simulink model "ProcessNetworkSimulation"  (R2015b)
settings: Solver=VariableStepAuto  StartTime=0.0  StopTime=1000.0  RelTol=1e-3
libraries: simulink x1, simeventslib x1
(part 17 of 21)

== system ProcessNetworkSimulation/Process_97 ==
  IN_Job : PathCombiner  NumberInputPorts=29
  OUT_Job : OutputSwitch  NumberOutputPorts=30  SwitchingCriterion=From attribute  AttributeName=outputFlowNode
  Process : Subsystem
  IN_Job_1 : PMIOPort  Port=1  Side=Left
  IN_Job_2 : PMIOPort  Port=2  Side=Left
  IN_Job_3 : PMIOPort  Port=3  Side=Left
  IN_Job_4 : PMIOPort  Port=4  Side=Left
  IN_Job_5 : PMIOPort  Port=5  Side=Left
  IN_Job_6 : PMIOPort  Port=6  Side=Left
  IN_Job_7 : PMIOPort  Port=7  Side=Left
  IN_Job_8 : PMIOPort  Port=8  Side=Left
  IN_Job_9 : PMIOPort  Port=9  Side=Left
  IN_Job_10 : PMIOPort  Port=10  Side=Left
  IN_Job_11 : PMIOPort  Port=11  Side=Left
  IN_Job_12 : PMIOPort  Port=12  Side=Left
  IN_Job_13 : PMIOPort  Port=13  Side=Left
  IN_Job_14 : PMIOPort  Port=14  Side=Left
  IN_Job_15 : PMIOPort  Port=15  Side=Left
  IN_Job_16 : PMIOPort  Port=16  Side=Left
  IN_Job_17 : PMIOPort  Port=17  Side=Left
  IN_Job_18 : PMIOPort  Port=18  Side=Left
  IN_Job_19 : PMIOPort  Port=19  Side=Left
  IN_Job_20 : PMIOPort  Port=20  Side=Left
  IN_Job_21 : PMIOPort  Port=21  Side=Left
  IN_Job_22 : PMIOPort  Port=22  Side=Left
  IN_Job_23 : PMIOPort  Port=23  Side=Left
  IN_Job_24 : PMIOPort  Port=24  Side=Left
  IN_Job_25 : PMIOPort  Port=25  Side=Left
  IN_Job_26 : PMIOPort  Port=26  Side=Left
  IN_Job_27 : PMIOPort  Port=27  Side=Left
  IN_Job_28 : PMIOPort  Port=28  Side=Left
  IN_Job_29 : PMIOPort  Port=29  Side=Left
  OUT_Job_1 : PMIOPort  Port=30  Side=Right
  OUT_Job_2 : PMIOPort  Port=31  Side=Right
  OUT_Job_3 : PMIOPort  Port=32  Side=Right
  OUT_Job_4 : PMIOPort  Port=33  Side=Right
  OUT_Job_5 : PMIOPort  Port=34  Side=Right
  OUT_Job_6 : PMIOPort  Port=35  Side=Right
  OUT_Job_7 : PMIOPort  Port=36  Side=Right
  OUT_Job_8 : PMIOPort  Port=37  Side=Right
  OUT_Job_9 : PMIOPort  Port=38  Side=Right
  OUT_Job_10 : PMIOPort  Port=39  Side=Right
  OUT_Job_11 : PMIOPort  Port=40  Side=Right
  OUT_Job_12 : PMIOPort  Port=41  Side=Right
  OUT_Job_13 : PMIOPort  Port=42  Side=Right
  OUT_Job_14 : PMIOPort  Port=43  Side=Right
  OUT_Job_15 : PMIOPort  Port=44  Side=Right
  OUT_Job_16 : PMIOPort  Port=45  Side=Right
  OUT_Job_17 : PMIOPort  Port=46  Side=Right
  OUT_Job_18 : PMIOPort  Port=47  Side=Right
  OUT_Job_19 : PMIOPort  Port=48  Side=Right
  OUT_Job_20 : PMIOPort  Port=49  Side=Right
  OUT_Job_21 : PMIOPort  Port=50  Side=Right
  OUT_Job_22 : PMIOPort  Port=51  Side=Right
  OUT_Job_23 : PMIOPort  Port=52  Side=Right
  OUT_Job_24 : PMIOPort  Port=53  Side=Right
  OUT_Job_25 : PMIOPort  Port=54  Side=Right
  OUT_Job_26 : PMIOPort  Port=55  Side=Right
  OUT_Job_27 : PMIOPort  Port=56  Side=Right
  OUT_Job_28 : PMIOPort  Port=57  Side=Right
  OUT_Job_29 : PMIOPort  Port=58  Side=Right
  OUT_Job_30 : PMIOPort  Port=59  Side=Right
  connections:
  OUT_Job/LConn1 -- Process/RConn1
  IN_Job/RConn1 -- Process/LConn1
  IN_Job/LConn1 -- IN_Job_1/RConn1
  IN_Job/LConn2 -- IN_Job_2/RConn1
  IN_Job/LConn3 -- IN_Job_3/RConn1
  IN_Job/LConn4 -- IN_Job_4/RConn1
  IN_Job/LConn5 -- IN_Job_5/RConn1
  IN_Job/LConn6 -- IN_Job_6/RConn1
  IN_Job/LConn7 -- IN_Job_7/RConn1
  IN_Job/LConn8 -- IN_Job_8/RConn1
  IN_Job/LConn9 -- IN_Job_9/RConn1
  IN_Job/LConn10 -- IN_Job_10/RConn1
  IN_Job/LConn11 -- IN_Job_11/RConn1
  IN_Job/LConn12 -- IN_Job_12/RConn1
  IN_Job/LConn13 -- IN_Job_13/RConn1
  IN_Job/LConn14 -- IN_Job_14/RConn1
  IN_Job/LConn15 -- IN_Job_15/RConn1
  IN_Job/LConn16 -- IN_Job_16/RConn1
  IN_Job/LConn17 -- IN_Job_17/RConn1
  IN_Job/LConn18 -- IN_Job_18/RConn1
  IN_Job/LConn19 -- IN_Job_19/RConn1
  IN_Job/LConn20 -- IN_Job_20/RConn1
  IN_Job/LConn21 -- IN_Job_21/RConn1
  IN_Job/LConn22 -- IN_Job_22/RConn1
  IN_Job/LConn23 -- IN_Job_23/RConn1
  IN_Job/LConn24 -- IN_Job_24/RConn1
  IN_Job/LConn25 -- IN_Job_25/RConn1
  IN_Job/LConn26 -- IN_Job_26/RConn1
  IN_Job/LConn27 -- IN_Job_27/RConn1
  IN_Job/LConn28 -- IN_Job_28/RConn1
  IN_Job/LConn29 -- IN_Job_29/RConn1
  OUT_Job/RConn1 -- OUT_Job_1/RConn1
  OUT_Job/RConn2 -- OUT_Job_2/RConn1
  OUT_Job/RConn3 -- OUT_Job_3/RConn1
  OUT_Job/RConn4 -- OUT_Job_4/RConn1
  OUT_Job/RConn5 -- OUT_Job_5/RConn1
  OUT_Job/RConn6 -- OUT_Job_6/RConn1
  OUT_Job/RConn7 -- OUT_Job_7/RConn1
  OUT_Job/RConn8 -- OUT_Job_8/RConn1
  OUT_Job/RConn9 -- OUT_Job_9/RConn1
  OUT_Job/RConn10 -- OUT_Job_10/RConn1
  OUT_Job/RConn11 -- OUT_Job_11/RConn1
  OUT_Job/RConn12 -- OUT_Job_12/RConn1
  OUT_Job/RConn13 -- OUT_Job_13/RConn1
  OUT_Job/RConn14 -- OUT_Job_14/RConn1
  OUT_Job/RConn15 -- OUT_Job_15/RConn1
  OUT_Job/RConn16 -- OUT_Job_16/RConn1
  OUT_Job/RConn17 -- OUT_Job_17/RConn1
  OUT_Job/RConn18 -- OUT_Job_18/RConn1
  OUT_Job/RConn19 -- OUT_Job_19/RConn1
  OUT_Job/RConn20 -- OUT_Job_20/RConn1
  OUT_Job/RConn21 -- OUT_Job_21/RConn1
  OUT_Job/RConn22 -- OUT_Job_22/RConn1
  OUT_Job/RConn23 -- OUT_Job_23/RConn1
  OUT_Job/RConn24 -- OUT_Job_24/RConn1
  OUT_Job/RConn25 -- OUT_Job_25/RConn1
  OUT_Job/RConn26 -- OUT_Job_26/RConn1
  OUT_Job/RConn27 -- OUT_Job_27/RConn1
  OUT_Job/RConn28 -- OUT_Job_28/RConn1
  OUT_Job/RConn29 -- OUT_Job_29/RConn1
  OUT_Job/RConn30 -- OUT_Job_30/RConn1

== system ProcessNetworkSimulation/Process_98 ==
  IN_Job : PathCombiner  NumberInputPorts=42
  OUT_Job : OutputSwitch  NumberOutputPorts=37  SwitchingCriterion=From attribute  AttributeName=outputFlowNode
  Process : Subsystem
  IN_Job_1 : PMIOPort  Port=1  Side=Left
  IN_Job_2 : PMIOPort  Port=2  Side=Left
  IN_Job_3 : PMIOPort  Port=3  Side=Left
  IN_Job_4 : PMIOPort  Port=4  Side=Left
  IN_Job_5 : PMIOPort  Port=5  Side=Left
  IN_Job_6 : PMIOPort  Port=6  Side=Left
  IN_Job_7 : PMIOPort  Port=7  Side=Left
  IN_Job_8 : PMIOPort  Port=8  Side=Left
  IN_Job_9 : PMIOPort  Port=9  Side=Left
  IN_Job_10 : PMIOPort  Port=10  Side=Left
  IN_Job_11 : PMIOPort  Port=11  Side=Left
  IN_Job_12 : PMIOPort  Port=12  Side=Left
  IN_Job_13 : PMIOPort  Port=13  Side=Left
  IN_Job_14 : PMIOPort  Port=14  Side=Left
  IN_Job_15 : PMIOPort  Port=15  Side=Left
  IN_Job_16 : PMIOPort  Port=16  Side=Left
  IN_Job_17 : PMIOPort  Port=17  Side=Left
  IN_Job_18 : PMIOPort  Port=18  Side=Left
  IN_Job_19 : PMIOPort  Port=19  Side=Left
  IN_Job_20 : PMIOPort  Port=20  Side=Left
  IN_Job_21 : PMIOPort  Port=21  Side=Left
  IN_Job_22 : PMIOPort  Port=22  Side=Left
  IN_Job_23 : PMIOPort  Port=23  Side=Left
  IN_Job_24 : PMIOPort  Port=24  Side=Left
  IN_Job_25 : PMIOPort  Port=25  Side=Left
  IN_Job_26 : PMIOPort  Port=26  Side=Left
  IN_Job_27 : PMIOPort  Port=27  Side=Left
  IN_Job_28 : PMIOPort  Port=28  Side=Left
  IN_Job_29 : PMIOPort  Port=29  Side=Left
  IN_Job_30 : PMIOPort  Port=30  Side=Left
  IN_Job_31 : PMIOPort  Port=31  Side=Left
  IN_Job_32 : PMIOPort  Port=32  Side=Left
  IN_Job_33 : PMIOPort  Port=33  Side=Left
  IN_Job_34 : PMIOPort  Port=34  Side=Left
  IN_Job_35 : PMIOPort  Port=35  Side=Left
  IN_Job_36 : PMIOPort  Port=36  Side=Left
  IN_Job_37 : PMIOPort  Port=37  Side=Left
  IN_Job_38 : PMIOPort  Port=38  Side=Left
  IN_Job_39 : PMIOPort  Port=39  Side=Left
  IN_Job_40 : PMIOPort  Port=40  Side=Left
  IN_Job_41 : PMIOPort  Port=41  Side=Left
  IN_Job_42 : PMIOPort  Port=42  Side=Left
  OUT_Job_1 : PMIOPort  Port=43  Side=Right
  OUT_Job_2 : PMIOPort  Port=44  Side=Right
  OUT_Job_3 : PMIOPort  Port=45  Side=Right
  OUT_Job_4 : PMIOPort  Port=46  Side=Right
  OUT_Job_5 : PMIOPort  Port=47  Side=Right
  OUT_Job_6 : PMIOPort  Port=48  Side=Right
  OUT_Job_7 : PMIOPort  Port=49  Side=Right
  OUT_Job_8 : PMIOPort  Port=50  Side=Right
  OUT_Job_9 : PMIOPort  Port=51  Side=Right
  OUT_Job_10 : PMIOPort  Port=52  Side=Right
  OUT_Job_11 : PMIOPort  Port=53  Side=Right
  OUT_Job_12 : PMIOPort  Port=54  Side=Right
  OUT_Job_13 : PMIOPort  Port=55  Side=Right
  OUT_Job_14 : PMIOPort  Port=56  Side=Right
  OUT_Job_15 : PMIOPort  Port=57  Side=Right
  OUT_Job_16 : PMIOPort  Port=58  Side=Right
  OUT_Job_17 : PMIOPort  Port=59  Side=Right
  OUT_Job_18 : PMIOPort  Port=60  Side=Right
  OUT_Job_19 : PMIOPort  Port=61  Side=Right
  OUT_Job_20 : PMIOPort  Port=62  Side=Right
  OUT_Job_21 : PMIOPort  Port=63  Side=Right
  OUT_Job_22 : PMIOPort  Port=64  Side=Right
  OUT_Job_23 : PMIOPort  Port=65  Side=Right
  OUT_Job_24 : PMIOPort  Port=66  Side=Right
  OUT_Job_25 : PMIOPort  Port=67  Side=Right
  OUT_Job_26 : PMIOPort  Port=68  Side=Right
  OUT_Job_27 : PMIOPort  Port=69  Side=Right
  OUT_Job_28 : PMIOPort  Port=70  Side=Right
  OUT_Job_29 : PMIOPort  Port=71  Side=Right
  OUT_Job_30 : PMIOPort  Port=72  Side=Right
  OUT_Job_31 : PMIOPort  Port=73  Side=Right
  OUT_Job_32 : PMIOPort  Port=74  Side=Right
  OUT_Job_33 : PMIOPort  Port=75  Side=Right
  OUT_Job_34 : PMIOPort  Port=76  Side=Right
  OUT_Job_35 : PMIOPort  Port=77  Side=Right
  OUT_Job_36 : PMIOPort  Port=78  Side=Right
  OUT_Job_37 : PMIOPort  Port=79  Side=Right
  connections:
  OUT_Job/LConn1 -- Process/RConn1
  IN_Job/RConn1 -- Process/LConn1
  IN_Job/LConn1 -- IN_Job_1/RConn1
  IN_Job/LConn2 -- IN_Job_2/RConn1
  IN_Job/LConn3 -- IN_Job_3/RConn1
  IN_Job/LConn4 -- IN_Job_4/RConn1
  IN_Job/LConn5 -- IN_Job_5/RConn1
  IN_Job/LConn6 -- IN_Job_6/RConn1
  IN_Job/LConn7 -- IN_Job_7/RConn1
  IN_Job/LConn8 -- IN_Job_8/RConn1
  IN_Job/LConn9 -- IN_Job_9/RConn1
  IN_Job/LConn10 -- IN_Job_10/RConn1
  IN_Job/LConn11 -- IN_Job_11/RConn1
  IN_Job/LConn12 -- IN_Job_12/RConn1
  IN_Job/LConn13 -- IN_Job_13/RConn1
  IN_Job/LConn14 -- IN_Job_14/RConn1
  IN_Job/LConn15 -- IN_Job_15/RConn1
  IN_Job/LConn16 -- IN_Job_16/RConn1
  IN_Job/LConn17 -- IN_Job_17/RConn1
  IN_Job/LConn18 -- IN_Job_18/RConn1
  IN_Job/LConn19 -- IN_Job_19/RConn1
  IN_Job/LConn20 -- IN_Job_20/RConn1
  IN_Job/LConn21 -- IN_Job_21/RConn1
  IN_Job/LConn22 -- IN_Job_22/RConn1
  IN_Job/LConn23 -- IN_Job_23/RConn1
  IN_Job/LConn24 -- IN_Job_24/RConn1
  IN_Job/LConn25 -- IN_Job_25/RConn1
  IN_Job/LConn26 -- IN_Job_26/RConn1
  IN_Job/LConn27 -- IN_Job_27/RConn1
  IN_Job/LConn28 -- IN_Job_28/RConn1
  IN_Job/LConn29 -- IN_Job_29/RConn1
  IN_Job/LConn30 -- IN_Job_30/RConn1
  IN_Job/LConn31 -- IN_Job_31/RConn1
  IN_Job/LConn32 -- IN_Job_32/RConn1
  IN_Job/LConn33 -- IN_Job_33/RConn1
  IN_Job/LConn34 -- IN_Job_34/RConn1
  IN_Job/LConn35 -- IN_Job_35/RConn1
  IN_Job/LConn36 -- IN_Job_36/RConn1
  IN_Job/LConn37 -- IN_Job_37/RConn1
  IN_Job/LConn38 -- IN_Job_38/RConn1
  IN_Job/LConn39 -- IN_Job_39/RConn1
  IN_Job/LConn40 -- IN_Job_40/RConn1
  IN_Job/LConn41 -- IN_Job_41/RConn1
  IN_Job/LConn42 -- IN_Job_42/RConn1
  OUT_Job/RConn1 -- OUT_Job_1/RConn1
  OUT_Job/RConn2 -- OUT_Job_2/RConn1
  OUT_Job/RConn3 -- OUT_Job_3/RConn1
  OUT_Job/RConn4 -- OUT_Job_4/RConn1
  OUT_Job/RConn5 -- OUT_Job_5/RConn1
  OUT_Job/RConn6 -- OUT_Job_6/RConn1
  OUT_Job/RConn7 -- OUT_Job_7/RConn1
  OUT_Job/RConn8 -- OUT_Job_8/RConn1
  OUT_Job/RConn9 -- OUT_Job_9/RConn1
  OUT_Job/RConn10 -- OUT_Job_10/RConn1
  OUT_Job/RConn11 -- OUT_Job_11/RConn1
  OUT_Job/RConn12 -- OUT_Job_12/RConn1
  OUT_Job/RConn13 -- OUT_Job_13/RConn1
  OUT_Job/RConn14 -- OUT_Job_14/RConn1
  OUT_Job/RConn15 -- OUT_Job_15/RConn1
  OUT_Job/RConn16 -- OUT_Job_16/RConn1
  OUT_Job/RConn17 -- OUT_Job_17/RConn1
  OUT_Job/RConn18 -- OUT_Job_18/RConn1
  OUT_Job/RConn19 -- OUT_Job_19/RConn1
  OUT_Job/RConn20 -- OUT_Job_20/RConn1
  OUT_Job/RConn21 -- OUT_Job_21/RConn1
  OUT_Job/RConn22 -- OUT_Job_22/RConn1
  OUT_Job/RConn23 -- OUT_Job_23/RConn1
  OUT_Job/RConn24 -- OUT_Job_24/RConn1
  OUT_Job/RConn25 -- OUT_Job_25/RConn1
  OUT_Job/RConn26 -- OUT_Job_26/RConn1
  OUT_Job/RConn27 -- OUT_Job_27/RConn1
  OUT_Job/RConn28 -- OUT_Job_28/RConn1
  OUT_Job/RConn29 -- OUT_Job_29/RConn1
  OUT_Job/RConn30 -- OUT_Job_30/RConn1
  OUT_Job/RConn31 -- OUT_Job_31/RConn1
  OUT_Job/RConn32 -- OUT_Job_32/RConn1
  OUT_Job/RConn33 -- OUT_Job_33/RConn1
  OUT_Job/RConn34 -- OUT_Job_34/RConn1
  OUT_Job/RConn35 -- OUT_Job_35/RConn1
  OUT_Job/RConn36 -- OUT_Job_36/RConn1
  OUT_Job/RConn37 -- OUT_Job_37/RConn1

== system ProcessNetworkSimulation/Process_99 ==
  IN_Job : PathCombiner  NumberInputPorts=46
  OUT_Job : OutputSwitch  NumberOutputPorts=40  SwitchingCriterion=From attribute  AttributeName=outputFlowNode
  Process : Subsystem
  IN_Job_1 : PMIOPort  Port=1  Side=Left
  IN_Job_2 : PMIOPort  Port=2  Side=Left
  IN_Job_3 : PMIOPort  Port=3  Side=Left
  IN_Job_4 : PMIOPort  Port=4  Side=Left
  IN_Job_5 : PMIOPort  Port=5  Side=Left
  IN_Job_6 : PMIOPort  Port=6  Side=Left
  IN_Job_7 : PMIOPort  Port=7  Side=Left
  IN_Job_8 : PMIOPort  Port=8  Side=Left
  IN_Job_9 : PMIOPort  Port=9  Side=Left
  IN_Job_10 : PMIOPort  Port=10  Side=Left
  IN_Job_11 : PMIOPort  Port=11  Side=Left
  IN_Job_12 : PMIOPort  Port=12  Side=Left
  IN_Job_13 : PMIOPort  Port=13  Side=Left
  IN_Job_14 : PMIOPort  Port=14  Side=Left
  IN_Job_15 : PMIOPort  Port=15  Side=Left
  IN_Job_16 : PMIOPort  Port=16  Side=Left
  IN_Job_17 : PMIOPort  Port=17  Side=Left
  IN_Job_18 : PMIOPort  Port=18  Side=Left
  IN_Job_19 : PMIOPort  Port=19  Side=Left
  IN_Job_20 : PMIOPort  Port=20  Side=Left
  IN_Job_21 : PMIOPort  Port=21  Side=Left
  IN_Job_22 : PMIOPort  Port=22  Side=Left
  IN_Job_23 : PMIOPort  Port=23  Side=Left
  IN_Job_24 : PMIOPort  Port=24  Side=Left
  IN_Job_25 : PMIOPort  Port=25  Side=Left
  IN_Job_26 : PMIOPort  Port=26  Side=Left
  IN_Job_27 : PMIOPort  Port=27  Side=Left
  IN_Job_28 : PMIOPort  Port=28  Side=Left
  IN_Job_29 : PMIOPort  Port=29  Side=Left
  IN_Job_30 : PMIOPort  Port=30  Side=Left
  IN_Job_31 : PMIOPort  Port=31  Side=Left
  IN_Job_32 : PMIOPort  Port=32  Side=Left
  IN_Job_33 : PMIOPort  Port=33  Side=Left
  IN_Job_34 : PMIOPort  Port=34  Side=Left
  IN_Job_35 : PMIOPort  Port=35  Side=Left
  IN_Job_36 : PMIOPort  Port=36  Side=Left
  IN_Job_37 : PMIOPort  Port=37  Side=Left
  IN_Job_38 : PMIOPort  Port=38  Side=Left
  IN_Job_39 : PMIOPort  Port=39  Side=Left
  IN_Job_40 : PMIOPort  Port=40  Side=Left
  IN_Job_41 : PMIOPort  Port=41  Side=Left
  IN_Job_42 : PMIOPort  Port=42  Side=Left
  IN_Job_43 : PMIOPort  Port=43  Side=Left
  IN_Job_44 : PMIOPort  Port=44  Side=Left
  IN_Job_45 : PMIOPort  Port=45  Side=Left
  IN_Job_46 : PMIOPort  Port=46  Side=Left
  OUT_Job_1 : PMIOPort  Port=47  Side=Right
  OUT_Job_2 : PMIOPort  Port=48  Side=Right
  OUT_Job_3 : PMIOPort  Port=49  Side=Right
  OUT_Job_4 : PMIOPort  Port=50  Side=Right
  OUT_Job_5 : PMIOPort  Port=51  Side=Right
  OUT_Job_6 : PMIOPort  Port=52  Side=Right
  OUT_Job_7 : PMIOPort  Port=53  Side=Right
  OUT_Job_8 : PMIOPort  Port=54  Side=Right
  OUT_Job_9 : PMIOPort  Port=55  Side=Right
  OUT_Job_10 : PMIOPort  Port=56  Side=Right
  OUT_Job_11 : PMIOPort  Port=57  Side=Right
  OUT_Job_12 : PMIOPort  Port=58  Side=Right
  OUT_Job_13 : PMIOPort  Port=59  Side=Right
  OUT_Job_14 : PMIOPort  Port=60  Side=Right
  OUT_Job_15 : PMIOPort  Port=61  Side=Right
  OUT_Job_16 : PMIOPort  Port=62  Side=Right
  OUT_Job_17 : PMIOPort  Port=63  Side=Right
  OUT_Job_18 : PMIOPort  Port=64  Side=Right
  OUT_Job_19 : PMIOPort  Port=65  Side=Right
  OUT_Job_20 : PMIOPort  Port=66  Side=Right
  OUT_Job_21 : PMIOPort  Port=67  Side=Right
  OUT_Job_22 : PMIOPort  Port=68  Side=Right
  OUT_Job_23 : PMIOPort  Port=69  Side=Right
  OUT_Job_24 : PMIOPort  Port=70  Side=Right
  OUT_Job_25 : PMIOPort  Port=71  Side=Right
  OUT_Job_26 : PMIOPort  Port=72  Side=Right
  OUT_Job_27 : PMIOPort  Port=73  Side=Right
  OUT_Job_28 : PMIOPort  Port=74  Side=Right
  OUT_Job_29 : PMIOPort  Port=75  Side=Right
  OUT_Job_30 : PMIOPort  Port=76  Side=Right
  OUT_Job_31 : PMIOPort  Port=77  Side=Right
  OUT_Job_32 : PMIOPort  Port=78  Side=Right
  OUT_Job_33 : PMIOPort  Port=79  Side=Right
  OUT_Job_34 : PMIOPort  Port=80  Side=Right
  OUT_Job_35 : PMIOPort  Port=81  Side=Right
  OUT_Job_36 : PMIOPort  Port=82  Side=Right
  OUT_Job_37 : PMIOPort  Port=83  Side=Right
  OUT_Job_38 : PMIOPort  Port=84  Side=Right
  OUT_Job_39 : PMIOPort  Port=85  Side=Right
  OUT_Job_40 : PMIOPort  Port=86  Side=Right
  connections:
  OUT_Job/LConn1 -- Process/RConn1
  IN_Job/RConn1 -- Process/LConn1
  IN_Job/LConn1 -- IN_Job_1/RConn1
  IN_Job/LConn2 -- IN_Job_2/RConn1
  IN_Job/LConn3 -- IN_Job_3/RConn1
  IN_Job/LConn4 -- IN_Job_4/RConn1
  IN_Job/LConn5 -- IN_Job_5/RConn1
  IN_Job/LConn6 -- IN_Job_6/RConn1
  IN_Job/LConn7 -- IN_Job_7/RConn1
  IN_Job/LConn8 -- IN_Job_8/RConn1
  IN_Job/LConn9 -- IN_Job_9/RConn1
  IN_Job/LConn10 -- IN_Job_10/RConn1
  IN_Job/LConn11 -- IN_Job_11/RConn1
  IN_Job/LConn12 -- IN_Job_12/RConn1
  IN_Job/LConn13 -- IN_Job_13/RConn1
  IN_Job/LConn14 -- IN_Job_14/RConn1
  IN_Job/LConn15 -- IN_Job_15/RConn1
  IN_Job/LConn16 -- IN_Job_16/RConn1
  IN_Job/LConn17 -- IN_Job_17/RConn1
  IN_Job/LConn18 -- IN_Job_18/RConn1
  IN_Job/LConn19 -- IN_Job_19/RConn1
  IN_Job/LConn20 -- IN_Job_20/RConn1
  IN_Job/LConn21 -- IN_Job_21/RConn1
  IN_Job/LConn22 -- IN_Job_22/RConn1
  IN_Job/LConn23 -- IN_Job_23/RConn1
  IN_Job/LConn24 -- IN_Job_24/RConn1
  IN_Job/LConn25 -- IN_Job_25/RConn1
  IN_Job/LConn26 -- IN_Job_26/RConn1
  IN_Job/LConn27 -- IN_Job_27/RConn1
  IN_Job/LConn28 -- IN_Job_28/RConn1
  IN_Job/LConn29 -- IN_Job_29/RConn1
  IN_Job/LConn30 -- IN_Job_30/RConn1
  IN_Job/LConn31 -- IN_Job_31/RConn1
  IN_Job/LConn32 -- IN_Job_32/RConn1
  IN_Job/LConn33 -- IN_Job_33/RConn1
  IN_Job/LConn34 -- IN_Job_34/RConn1
  IN_Job/LConn35 -- IN_Job_35/RConn1
  IN_Job/LConn36 -- IN_Job_36/RConn1
  IN_Job/LConn37 -- IN_Job_37/RConn1
  IN_Job/LConn38 -- IN_Job_38/RConn1
  IN_Job/LConn39 -- IN_Job_39/RConn1
  IN_Job/LConn40 -- IN_Job_40/RConn1
  IN_Job/LConn41 -- IN_Job_41/RConn1
  IN_Job/LConn42 -- IN_Job_42/RConn1
  IN_Job/LConn43 -- IN_Job_43/RConn1
  IN_Job/LConn44 -- IN_Job_44/RConn1
  IN_Job/LConn45 -- IN_Job_45/RConn1
  IN_Job/LConn46 -- IN_Job_46/RConn1
  OUT_Job/RConn1 -- OUT_Job_1/RConn1
  OUT_Job/RConn2 -- OUT_Job_2/RConn1
  OUT_Job/RConn3 -- OUT_Job_3/RConn1
  OUT_Job/RConn4 -- OUT_Job_4/RConn1
  OUT_Job/RConn5 -- OUT_Job_5/RConn1
  OUT_Job/RConn6 -- OUT_Job_6/RConn1
  OUT_Job/RConn7 -- OUT_Job_7/RConn1
  OUT_Job/RConn8 -- OUT_Job_8/RConn1
  OUT_Job/RConn9 -- OUT_Job_9/RConn1
  OUT_Job/RConn10 -- OUT_Job_10/RConn1
  OUT_Job/RConn11 -- OUT_Job_11/RConn1
  OUT_Job/RConn12 -- OUT_Job_12/RConn1
  OUT_Job/RConn13 -- OUT_Job_13/RConn1
  OUT_Job/RConn14 -- OUT_Job_14/RConn1
  OUT_Job/RConn15 -- OUT_Job_15/RConn1
  OUT_Job/RConn16 -- OUT_Job_16/RConn1
  OUT_Job/RConn17 -- OUT_Job_17/RConn1
  OUT_Job/RConn18 -- OUT_Job_18/RConn1
  OUT_Job/RConn19 -- OUT_Job_19/RConn1
  OUT_Job/RConn20 -- OUT_Job_20/RConn1
  OUT_Job/RConn21 -- OUT_Job_21/RConn1
  OUT_Job/RConn22 -- OUT_Job_22/RConn1
  OUT_Job/RConn23 -- OUT_Job_23/RConn1
  OUT_Job/RConn24 -- OUT_Job_24/RConn1
  OUT_Job/RConn25 -- OUT_Job_25/RConn1
  OUT_Job/RConn26 -- OUT_Job_26/RConn1
  OUT_Job/RConn27 -- OUT_Job_27/RConn1
  OUT_Job/RConn28 -- OUT_Job_28/RConn1
  OUT_Job/RConn29 -- OUT_Job_29/RConn1
  OUT_Job/RConn30 -- OUT_Job_30/RConn1
  OUT_Job/RConn31 -- OUT_Job_31/RConn1
  OUT_Job/RConn32 -- OUT_Job_32/RConn1
  OUT_Job/RConn33 -- OUT_Job_33/RConn1
  OUT_Job/RConn34 -- OUT_Job_34/RConn1
  OUT_Job/RConn35 -- OUT_Job_35/RConn1
  OUT_Job/RConn36 -- OUT_Job_36/RConn1
  OUT_Job/RConn37 -- OUT_Job_37/RConn1
  OUT_Job/RConn38 -- OUT_Job_38/RConn1
  OUT_Job/RConn39 -- OUT_Job_39/RConn1
  OUT_Job/RConn40 -- OUT_Job_40/RConn1

== system ProcessNetworkSimulation/Arrival_Process/Process ==
  ProcessQueue : FIFOQueue  Capacity=Inf  StatAverageWait=on  StatAverageQueueLength=on
      settings: OutputPortMap=o2,o3
  ProcessServer : NServer  NumberOfServers=Inf  ServiceTime=0  StatNumberDeparted=on  StatUtilization=on
      settings: OutputPortMap=o0,o5
  ProcessTime : EventBasedRandomNumber  meanExp=0.0075758  minUnif=1  meanNorm=2  stdNorm=0.2  Seed=42055
  Routing : EventBasedRandomNumber  Distribution=Arbitrary discrete  valueVecDisc=[0,1,2,3,4,5,6,7,8,9,10,11,12,13,14,15,16,17,18,19,20,21,22,23,24,25,26,27,28,29,30,31,32,33,34,35,36,37,38,39,40,41,42,43,44,45,46,47,48,49,50,51,52,53,54,55,56,57,58,59,60,61,62,63,64,65,66,67,68,69,70,71,72,73,74,75,76,77,78,79,80,81,82,83,84,85,86,87,88,89,90,91,92,93,94,95,96,97,98,99,100]  probVecDisc=[0,0,0,0,0.0152,0,0,0,0,0,0.0076,0,0,0.0152,0,0.0455,0.053,0,0,0,0,0,0,0,0,0,0,0,0.0379,0,0,0,0,0,0,0,0,0,0,0,0,0,0,0.0682,0,0,0,0,0,0.053,0,0,0,0,0,0.0682,0,0,0,0,0,0,0,0,0.053,0,0.0682,0,0,0,0,0,0,0,0,0,0,0,0,0,0.0606,0.0227,0.0379,0,0,0.0152,0,0,0,0,0,0.053,0.0909,0,0.0152,0,0.1589,0.0379,0.0227,0,0]  Seed=45272
  arrivalGenerator : TimeBasedEntityGenerator  GenerateEntitiesUpon=Intergeneration time from port t
  read_ProcessTimer : ReadTimer  TimerTag=T_Arrival_Process  StatAverageTimeElapsed=on
      settings: OutputPortMap=o3
  setRouting : SetAttribute  AttributeName=outputFlowNode  AttributeFrom=Signal port  EvaluatedAttributeValue={ []}
  start_ProcessTimer : StartTimer  TimerTag=T_Arrival_Process  TimerStartedOption=Restart
  OUT_Job : PMIOPort  Port=1  Side=Right
  wires:
  Routing/1 -> setRouting/1
  ProcessTime/1 -> arrivalGenerator/1
  connections:
  ProcessServer/RConn1 -- setRouting/LConn1
  setRouting/RConn1 -- OUT_Job/RConn1
  arrivalGenerator/RConn1 -- ProcessQueue/LConn1
  start_ProcessTimer/RConn1 -- read_ProcessTimer/LConn1
  ProcessQueue/RConn1 -- ProcessServer/LConn1

== system ProcessNetworkSimulation/Departure_Process/Process ==
  Compare To Constant : simulink/Logic and Bit Operations/Compare To Constant  relop=>=  const=1000  OutDataTypeStr=boolean
  Discrete Event Signal to Workspace : simeventslib/SimEvents Sinks/Discrete Event Signal to Workspace  VariableName=ProcessTime  SaveFormat=Structure With Time  isMonitorOnly=off  isRecordIC=off
  Entity Sink : EntitySink  StatNumberArrived=on
  Event to Timed Signal : EventToTimedSignal
  ProcessQueue : FIFOQueue  Capacity=Inf  StatAverageWait=on  StatAverageQueueLength=on
      settings: OutputPortMap=o2,o3
  ProcessServer : NServer  NumberOfServers=Inf  ServiceTimeFrom=Signal port t  StatNumberDeparted=on  StatUtilization=on
      settings: OutputPortMap=o0,o5
  ProcessTime : EventBasedRandomNumber  Distribution=Gaussian (normal)  minUnif=1  stdNorm=2.2204e-16  Seed=48489
  Routing : EventBasedRandomNumber  Distribution=Arbitrary discrete  valueVecDisc=[0,1,2]  probVecDisc=[0,1,0]  Seed=51706
  Stop Simulation : Stop
  SystemTimer : ReadTimer  TimerTag=T_LHS_BU_1  StatTimeElapsed=on
      settings: OutputPortMap=o2
  read_ProcessTimer : ReadTimer  TimerTag=T_Departure_Process  StatAverageTimeElapsed=on
      settings: OutputPortMap=o3
  setRouting : SetAttribute  AttributeName=outputFlowNode  AttributeFrom=Signal port  EvaluatedAttributeValue={ []}
  start_ProcessTimer : StartTimer  TimerTag=T_Departure_Process  TimerStartedOption=Restart
  IN_Job : PMIOPort  Port=1  Side=Left
  wires:
  ProcessTime/1 -> ProcessServer/1
  Routing/1 -> setRouting/1
  Entity Sink/1 -> Event to Timed Signal/1
  Event to Timed Signal/1 -> Compare To Constant/1
  Compare To Constant/1 -> Stop Simulation/1
  SystemTimer/1 -> Discrete Event Signal to Workspace/1
  connections:
  IN_Job/RConn1 -- ProcessQueue/LConn1
  ProcessServer/RConn1 -- SystemTimer/LConn1
  ProcessQueue/RConn1 -- ProcessServer/LConn1
  SystemTimer/RConn1 -- Entity Sink/LConn1
  start_ProcessTimer/RConn1 -- read_ProcessTimer/LConn1

== system ProcessNetworkSimulation/Process_1/Process ==
  OUTQueue : FIFOQueue  Capacity=inf
  ProcessQueue : FIFOQueue  Capacity=Inf  StatAverageWait=on  StatAverageQueueLength=on
      settings: OutputPortMap=o2,o3
  ProcessServer : NServer  NumberOfServers=9  ServiceTimeFrom=Signal port t  StatNumberDeparted=on  StatUtilization=on
      settings: OutputPortMap=o0,o5
  ProcessTime : EventBasedRandomNumber  meanExp=0.05  minUnif=1  meanNorm=2  stdNorm=0.2  Seed=54923
  Routing : EventBasedRandomNumber  Distribution=Arbitrary discrete  valueVecDisc=[0,1,2,3,4,5,6,7,8,9,10,11,12,13,14,15,16,17,18,19,20,21,22,23,24,25,26,27,28,29,30,31,32,33,34,35,36,37]  probVecDisc=[0,0.0106,0.0319,0.0106,0.0372,0.0106,0.0266,0.0536,0.0106,0.0106,0.0106,0.0319,0.0319,0.016,0.016,0.0372,0.0372,0.0479,0.0266,0.0106,0.0372,0.0479,0.0319,0.0319,0.0106,0.0106,0.0106,0.0479,0.0479,0.0053,0.0319,0.0479,0.0532,0.0106,0.0479,0.0319,0.0266,0]  Seed=58140
  read_ProcessTimer : ReadTimer  TimerTag=T_Process_1  StatAverageTimeElapsed=on
      settings: OutputPortMap=o3
  setRouting : SetAttribute  AttributeName=outputFlowNode  AttributeFrom=Signal port  EvaluatedAttributeValue={ []}
  start_ProcessTimer : StartTimer  TimerTag=T_Process_1  TimerStartedOption=Restart
  IN_Job : PMIOPort  Port=1  Side=Left
  OUT_Job : PMIOPort  Port=2  Side=Right
  wires:
  Routing/1 -> setRouting/1
  ProcessTime/1 -> ProcessServer/1
  connections:
  setRouting/LConn1 -- OUTQueue/RConn1
  IN_Job/RConn1 -- start_ProcessTimer/LConn1
  ProcessServer/RConn1 -- read_ProcessTimer/LConn1
  start_ProcessTimer/RConn1 -- ProcessQueue/LConn1
  ProcessQueue/RConn1 -- ProcessServer/LConn1
  read_ProcessTimer/RConn1 -- OUTQueue/LConn1
  OUT_Job/RConn1 -- setRouting/RConn1

== system ProcessNetworkSimulation/Process_10/Process ==
  OUTQueue : FIFOQueue  Capacity=inf
  ProcessQueue : FIFOQueue  Capacity=Inf  StatAverageWait=on  StatAverageQueueLength=on
      settings: OutputPortMap=o2,o3
  ProcessServer : NServer  NumberOfServers=13  ServiceTimeFrom=Signal port t  StatNumberDeparted=on  StatUtilization=on
      settings: OutputPortMap=o0,o5
  ProcessTime : EventBasedRandomNumber  meanExp=0.05  minUnif=1  meanNorm=2  stdNorm=0.2  Seed=61357
  Routing : EventBasedRandomNumber  Distribution=Arbitrary discrete  valueVecDisc=[0,1,2,3,4,5,6,7,8,9,10,11,12,13,14,15,16,17,18,19,20,21,22,23,24,25,26,27,28,29,30,31,32,33,34,35,36,37,38,39,40,41]  probVecDisc=[0,0.0246,0.0365,0.0287,0.0369,0.0246,0.0369,0.0328,0.0041,0.0082,0.0369,0.0287,0.0328,0.0328,0.0205,0.0246,0.0287,0.0287,0.0287,0.0082,0.0369,0.0205,0.0287,0.0287,0.0246,0.0123,0.0041,0.0082,0.0246,0.0246,0.0369,0.0246,0.0123,0.0369,0.0369,0.0082,0.0205,0.0369,0.0205,0.0123,0.0369,0]  Seed=64574
  read_ProcessTimer : ReadTimer  TimerTag=T_Process_10  StatAverageTimeElapsed=on
      settings: OutputPortMap=o3
  setRouting : SetAttribute  AttributeName=outputFlowNode  AttributeFrom=Signal port  EvaluatedAttributeValue={ []}
  start_ProcessTimer : StartTimer  TimerTag=T_Process_10  TimerStartedOption=Restart
  IN_Job : PMIOPort  Port=1  Side=Left
  OUT_Job : PMIOPort  Port=2  Side=Right
  wires:
  Routing/1 -> setRouting/1
  ProcessTime/1 -> ProcessServer/1
  connections:
  setRouting/LConn1 -- OUTQueue/RConn1
  IN_Job/RConn1 -- start_ProcessTimer/LConn1
  ProcessServer/RConn1 -- read_ProcessTimer/LConn1
  start_ProcessTimer/RConn1 -- ProcessQueue/LConn1
  ProcessQueue/RConn1 -- ProcessServer/LConn1
  read_ProcessTimer/RConn1 -- OUTQueue/LConn1
  OUT_Job/RConn1 -- setRouting/RConn1

== system ProcessNetworkSimulation/Process_100/Process ==
  OUTQueue : FIFOQueue  Capacity=inf
  ProcessQueue : FIFOQueue  Capacity=Inf  StatAverageWait=on  StatAverageQueueLength=on
      settings: OutputPortMap=o2,o3
  ProcessServer : NServer  NumberOfServers=10  ServiceTimeFrom=Signal port t  StatNumberDeparted=on  StatUtilization=on
      settings: OutputPortMap=o0,o5
  ProcessTime : EventBasedRandomNumber  meanExp=0.05  minUnif=1  meanNorm=2  stdNorm=0.2  Seed=2255
  Routing : EventBasedRandomNumber  Distribution=Arbitrary discrete  valueVecDisc=[0,1,2,3,4,5,6,7,8,9,10,11,12,13,14,15,16,17,18,19,20,21,22,23,24,25,26,27,28,29,30]  probVecDisc=[0,0.0467,0.0133,0.02,0.0133,0.067,0.0333,0.0467,0.0133,0.04,0.02,0.04,0.0533,0.06,0.0333,0.02,0.0467,0.0133,0.0133,0.02,0.0133,0.0133,0.0533,0.0133,0.0333,0.0667,0.04,0.04,0.06,0.0533,0]  Seed=5472
  read_ProcessTimer : ReadTimer  TimerTag=T_Process_100  StatAverageTimeElapsed=on
      settings: OutputPortMap=o3
  setRouting : SetAttribute  AttributeName=outputFlowNode  AttributeFrom=Signal port  EvaluatedAttributeValue={ []}
  start_ProcessTimer : StartTimer  TimerTag=T_Process_100  TimerStartedOption=Restart
  IN_Job : PMIOPort  Port=1  Side=Left
  OUT_Job : PMIOPort  Port=2  Side=Right
  wires:
  Routing/1 -> setRouting/1
  ProcessTime/1 -> ProcessServer/1
  connections:
  setRouting/LConn1 -- OUTQueue/RConn1
  IN_Job/RConn1 -- start_ProcessTimer/LConn1
  ProcessServer/RConn1 -- read_ProcessTimer/LConn1
  start_ProcessTimer/RConn1 -- ProcessQueue/LConn1
  ProcessQueue/RConn1 -- ProcessServer/LConn1
  read_ProcessTimer/RConn1 -- OUTQueue/LConn1
  OUT_Job/RConn1 -- setRouting/RConn1

== system ProcessNetworkSimulation/Process_11/Process ==
  OUTQueue : FIFOQueue  Capacity=inf
  ProcessQueue : FIFOQueue  Capacity=Inf  StatAverageWait=on  StatAverageQueueLength=on
      settings: OutputPortMap=o2,o3
  ProcessServer : NServer  NumberOfServers=12  ServiceTimeFrom=Signal port t  StatNumberDeparted=on  StatUtilization=on
      settings: OutputPortMap=o0,o5
  ProcessTime : EventBasedRandomNumber  meanExp=0.05  minUnif=1  meanNorm=2  stdNorm=0.2  Seed=8689
  Routing : EventBasedRandomNumber  Distribution=Arbitrary discrete  valueVecDisc=[0,1,2,3,4,5,6,7,8,9,10,11,12,13,14,15,16,17,18,19,20,21,22,23,24,25,26,27,28,29,30,31,32,33,34,35,36,37]  probVecDisc=[0,0.0105,0.0158,0.0105,0.0316,0.0368,0.0105,0.0105,0.0421,0.0528,0.0263,0.0158,0.0316,0.0474,0.0105,0.0368,0.0053,0.0421,0.0263,0.0474,0.0158,0.0105,0.0158,0.0105,0.0368,0.0474,0.0526,0.0105,0.0368,0.0474,0.0316,0.0053,0.0158,0.0316,0.0316,0.0526,0.0368,0]  Seed=11906
  read_ProcessTimer : ReadTimer  TimerTag=T_Process_11  StatAverageTimeElapsed=on
      settings: OutputPortMap=o3
  setRouting : SetAttribute  AttributeName=outputFlowNode  AttributeFrom=Signal port  EvaluatedAttributeValue={ []}
  start_ProcessTimer : StartTimer  TimerTag=T_Process_11  TimerStartedOption=Restart
  IN_Job : PMIOPort  Port=1  Side=Left
  OUT_Job : PMIOPort  Port=2  Side=Right
  wires:
  Routing/1 -> setRouting/1
  ProcessTime/1 -> ProcessServer/1
  connections:
  setRouting/LConn1 -- OUTQueue/RConn1
  IN_Job/RConn1 -- start_ProcessTimer/LConn1
  ProcessServer/RConn1 -- read_ProcessTimer/LConn1
  start_ProcessTimer/RConn1 -- ProcessQueue/LConn1
  ProcessQueue/RConn1 -- ProcessServer/LConn1
  read_ProcessTimer/RConn1 -- OUTQueue/LConn1
  OUT_Job/RConn1 -- setRouting/RConn1

== system ProcessNetworkSimulation/Process_12/Process ==
  OUTQueue : FIFOQueue  Capacity=inf
  ProcessQueue : FIFOQueue  Capacity=Inf  StatAverageWait=on  StatAverageQueueLength=on
      settings: OutputPortMap=o2,o3
  ProcessServer : NServer  NumberOfServers=11  ServiceTimeFrom=Signal port t  StatNumberDeparted=on  StatUtilization=on
      settings: OutputPortMap=o0,o5
  ProcessTime : EventBasedRandomNumber  meanExp=0.05  minUnif=1  meanNorm=2  stdNorm=0.2  Seed=15123
  Routing : EventBasedRandomNumber  Distribution=Arbitrary discrete  valueVecDisc=[0,1,2,3,4,5,6,7,8,9,10,11,12,13,14,15,16,17,18,19,20,21,22,23,24,25,26,27,28,29,30,31,32,33,34,35,36,37,38,39,40,41]  probVecDisc=[0,0.0313,0.0089,0.0223,0.0313,0.0089,0.0223,0.0357,0.0089,0.0268,0.0268,0.0445,0.0134,0.0134,0.0089,0.0089,0.0045,0.0402,0.0223,0.0313,0.0402,0.0089,0.0134,0.0134,0.0268,0.0223,0.0045,0.0223,0.0402,0.0089,0.0223,0.0357,0.0313,0.0402,0.0402,0.0223,0.0313,0.0446,0.0402,0.0402,0.0402,0]  Seed=18340
  read_ProcessTimer : ReadTimer  TimerTag=T_Process_12  StatAverageTimeElapsed=on
      settings: OutputPortMap=o3
  setRouting : SetAttribute  AttributeName=outputFlowNode  AttributeFrom=Signal port  EvaluatedAttributeValue={ []}
  start_ProcessTimer : StartTimer  TimerTag=T_Process_12  TimerStartedOption=Restart
  IN_Job : PMIOPort  Port=1  Side=Left
  OUT_Job : PMIOPort  Port=2  Side=Right
  wires:
  Routing/1 -> setRouting/1
  ProcessTime/1 -> ProcessServer/1
  connections:
  setRouting/LConn1 -- OUTQueue/RConn1
  IN_Job/RConn1 -- start_ProcessTimer/LConn1
  ProcessServer/RConn1 -- read_ProcessTimer/LConn1
  start_ProcessTimer/RConn1 -- ProcessQueue/LConn1
  ProcessQueue/RConn1 -- ProcessServer/LConn1
  read_ProcessTimer/RConn1 -- OUTQueue/LConn1
  OUT_Job/RConn1 -- setRouting/RConn1

== system ProcessNetworkSimulation/Process_13/Process ==
  OUTQueue : FIFOQueue  Capacity=inf
  ProcessQueue : FIFOQueue  Capacity=Inf  StatAverageWait=on  StatAverageQueueLength=on
      settings: OutputPortMap=o2,o3
  ProcessServer : NServer  NumberOfServers=13  ServiceTimeFrom=Signal port t  StatNumberDeparted=on  StatUtilization=on
      settings: OutputPortMap=o0,o5
  ProcessTime : EventBasedRandomNumber  meanExp=0.05  minUnif=1  meanNorm=2  stdNorm=0.2  Seed=21557
  Routing : EventBasedRandomNumber  Distribution=Arbitrary discrete  valueVecDisc=[0,1,2,3,4,5,6,7,8,9,10,11,12,13,14,15,16,17,18,19,20,21,22,23,24,25,26,27,28,29,30,31,32,33,34,35,36,37,38,39,40,41,42]  probVecDisc=[0,0.0093,0.0374,0.0234,0.028,0.028,0.028,0.0327,0.0327,0.014,0.028,0.014,0.0327,0.0093,0.0327,0.0093,0.0234,0.028,0.0421,0.0093,0.0421,0.0093,0.0421,0.0421,0.028,0.014,0.0093,0.014,0.0093,0.0327,0.0327,0.0421,0.014,0.0093,0.0421,0.014,0.028,0.0093,0.0374,0.0093,0.0093,0.0473,0]  Seed=24774
  read_ProcessTimer : ReadTimer  TimerTag=T_Process_13  StatAverageTimeElapsed=on
      settings: OutputPortMap=o3
  setRouting : SetAttribute  AttributeName=outputFlowNode  AttributeFrom=Signal port  EvaluatedAttributeValue={ []}
  start_ProcessTimer : StartTimer  TimerTag=T_Process_13  TimerStartedOption=Restart
  IN_Job : PMIOPort  Port=1  Side=Left
  OUT_Job : PMIOPort  Port=2  Side=Right
  wires:
  Routing/1 -> setRouting/1
  ProcessTime/1 -> ProcessServer/1
  connections:
  setRouting/LConn1 -- OUTQueue/RConn1
  IN_Job/RConn1 -- start_ProcessTimer/LConn1
  ProcessServer/RConn1 -- read_ProcessTimer/LConn1
  start_ProcessTimer/RConn1 -- ProcessQueue/LConn1
  ProcessQueue/RConn1 -- ProcessServer/LConn1
  read_ProcessTimer/RConn1 -- OUTQueue/LConn1
  OUT_Job/RConn1 -- setRouting/RConn1

== system ProcessNetworkSimulation/Process_14/Process ==
  OUTQueue : FIFOQueue  Capacity=inf
  ProcessQueue : FIFOQueue  Capacity=Inf  StatAverageWait=on  StatAverageQueueLength=on
      settings: OutputPortMap=o2,o3
  ProcessServer : NServer  NumberOfServers=12  ServiceTimeFrom=Signal port t  StatNumberDeparted=on  StatUtilization=on
      settings: OutputPortMap=o0,o5
  ProcessTime : EventBasedRandomNumber  meanExp=0.05  minUnif=1  meanNorm=2  stdNorm=0.2  Seed=27991
  Routing : EventBasedRandomNumber  Distribution=Arbitrary discrete  valueVecDisc=[0,1,2,3,4,5,6,7,8,9,10,11,12,13,14,15,16,17,18,19,20,21,22,23,24,25,26,27,28,29,30,31,32,33,34,35,36,37,38,39,40]  probVecDisc=[0,0.0238,0.0095,0.0048,0.0333,0.0095,0.0381,0.0143,0.0429,0.0238,0.0238,0.0238,0.0429,0.0429,0.0429,0.0381,0.0333,0.0286,0.0429,0.0286,0.0381,0.0333,0.0095,0.0333,0.0095,0.0381,0.0095,0.0286,0.0143,0.0095,0.0095,0.0429,0.0476,0.0095,0.0095,0.0333,0.0286,0.0286,0.0095,0.0095,0]  Seed=31208
  read_ProcessTimer : ReadTimer  TimerTag=T_Process_14  StatAverageTimeElapsed=on
      settings: OutputPortMap=o3
  setRouting : SetAttribute  AttributeName=outputFlowNode  AttributeFrom=Signal port  EvaluatedAttributeValue={ []}
  start_ProcessTimer : StartTimer  TimerTag=T_Process_14  TimerStartedOption=Restart
  IN_Job : PMIOPort  Port=1  Side=Left
  OUT_Job : PMIOPort  Port=2  Side=Right
  wires:
  Routing/1 -> setRouting/1
  ProcessTime/1 -> ProcessServer/1
  connections:
  setRouting/LConn1 -- OUTQueue/RConn1
  IN_Job/RConn1 -- start_ProcessTimer/LConn1
  ProcessServer/RConn1 -- read_ProcessTimer/LConn1
  start_ProcessTimer/RConn1 -- ProcessQueue/LConn1
  ProcessQueue/RConn1 -- ProcessServer/LConn1
  read_ProcessTimer/RConn1 -- OUTQueue/LConn1
  OUT_Job/RConn1 -- setRouting/RConn1

== system ProcessNetworkSimulation/Process_15/Process ==
  OUTQueue : FIFOQueue  Capacity=inf
  ProcessQueue : FIFOQueue  Capacity=Inf  StatAverageWait=on  StatAverageQueueLength=on
      settings: OutputPortMap=o2,o3
  ProcessServer : NServer  NumberOfServers=12  ServiceTimeFrom=Signal port t  StatNumberDeparted=on  StatUtilization=on
      settings: OutputPortMap=o0,o5
  ProcessTime : EventBasedRandomNumber  meanExp=0.05  minUnif=1  meanNorm=2  stdNorm=0.2  Seed=34425
  Routing : EventBasedRandomNumber  Distribution=Arbitrary discrete  valueVecDisc=[0,1,2,3,4,5,6,7,8,9,10,11,12,13,14,15,16,17,18,19,20,21,22,23,24,25,26,27,28,29,30,31,32,33,34,35,36,37,38]  probVecDisc=[0,0.0102,0.0305,0.0102,0.0355,0.0102,0.0102,0.0152,0.0102,0.0457,0.0051,0.0152,0.0457,0.0355,0.0457,0.0305,0.0102,0.0355,0.0305,0.0152,0.0457,0.0305,0.0355,0.0406,0.0457,0.0355,0.0254,0.0355,0.0457,0.0305,0.0305,0.0102,0.0152,0.0152,0.0152,0.0504,0.0355,0.0102,0]  Seed=37642
  read_ProcessTimer : ReadTimer  TimerTag=T_Process_15  StatAverageTimeElapsed=on
      settings: OutputPortMap=o3
  setRouting : SetAttribute  AttributeName=outputFlowNode  AttributeFrom=Signal port  EvaluatedAttributeValue={ []}
  start_ProcessTimer : StartTimer  TimerTag=T_Process_15  TimerStartedOption=Restart
  IN_Job : PMIOPort  Port=1  Side=Left
  OUT_Job : PMIOPort  Port=2  Side=Right
  wires:
  Routing/1 -> setRouting/1
  ProcessTime/1 -> ProcessServer/1
  connections:
  setRouting/LConn1 -- OUTQueue/RConn1
  IN_Job/RConn1 -- start_ProcessTimer/LConn1
  ProcessServer/RConn1 -- read_ProcessTimer/LConn1
  start_ProcessTimer/RConn1 -- ProcessQueue/LConn1
  ProcessQueue/RConn1 -- ProcessServer/LConn1
  read_ProcessTimer/RConn1 -- OUTQueue/LConn1
  OUT_Job/RConn1 -- setRouting/RConn1

== system ProcessNetworkSimulation/Process_16/Process ==
  OUTQueue : FIFOQueue  Capacity=inf
  ProcessQueue : FIFOQueue  Capacity=Inf  StatAverageWait=on  StatAverageQueueLength=on
      settings: OutputPortMap=o2,o3
  ProcessServer : NServer  NumberOfServers=12  ServiceTimeFrom=Signal port t  StatNumberDeparted=on  StatUtilization=on
      settings: OutputPortMap=o0,o5
  ProcessTime : EventBasedRandomNumber  meanExp=0.05  minUnif=1  meanNorm=2  stdNorm=0.2  Seed=40859
  Routing : EventBasedRandomNumber  Distribution=Arbitrary discrete  valueVecDisc=[0,1,2,3,4,5,6,7,8,9,10,11,12,13,14,15,16,17,18,19,20,21,22,23,24,25,26,27,28,29,30,31,32,33,34,35,36,37,38,39,40]  probVecDisc=[0,0.009,0.0135,0.0225,0.0315,0.0405,0.0405,0.009,0.0135,0.0405,0.0135,0.046,0.0135,0.0405,0.027,0.0135,0.0225,0.027,0.009,0.0405,0.045,0.036,0.027,0.0315,0.0045,0.0405,0.009,0.0405,0.009,0.009,0.027,0.0315,0.0225,0.027,0.009,0.009,0.0405,0.027,0.0405,0.0405,0]  Seed=44076
  read_ProcessTimer : ReadTimer  TimerTag=T_Process_16  StatAverageTimeElapsed=on
      settings: OutputPortMap=o3
  setRouting : SetAttribute  AttributeName=outputFlowNode  AttributeFrom=Signal port  EvaluatedAttributeValue={ []}
  start_ProcessTimer : StartTimer  TimerTag=T_Process_16  TimerStartedOption=Restart
  IN_Job : PMIOPort  Port=1  Side=Left
  OUT_Job : PMIOPort  Port=2  Side=Right
  wires:
  Routing/1 -> setRouting/1
  ProcessTime/1 -> ProcessServer/1
  connections:
  setRouting/LConn1 -- OUTQueue/RConn1
  IN_Job/RConn1 -- start_ProcessTimer/LConn1
  ProcessServer/RConn1 -- read_ProcessTimer/LConn1
  start_ProcessTimer/RConn1 -- ProcessQueue/LConn1
  ProcessQueue/RConn1 -- ProcessServer/LConn1
  read_ProcessTimer/RConn1 -- OUTQueue/LConn1
  OUT_Job/RConn1 -- setRouting/RConn1

== system ProcessNetworkSimulation/Process_17/Process ==
  OUTQueue : FIFOQueue  Capacity=inf
  ProcessQueue : FIFOQueue  Capacity=Inf  StatAverageWait=on  StatAverageQueueLength=on
      settings: OutputPortMap=o2,o3
  ProcessServer : NServer  NumberOfServers=11  ServiceTimeFrom=Signal port t  StatNumberDeparted=on  StatUtilization=on
      settings: OutputPortMap=o0,o5
  ProcessTime : EventBasedRandomNumber  meanExp=0.05  minUnif=1  meanNorm=2  stdNorm=0.2  Seed=47293
  Routing : EventBasedRandomNumber  Distribution=Arbitrary discrete  valueVecDisc=[0,1,2,3,4,5,6,7,8,9,10,11,12,13,14,15,16,17,18,19,20,21,22,23,24,25,26,27,28,29,30,31,32,33]  probVecDisc=[0,0.012,0.012,0.0181,0.0181,0.0181,0.0181,0.0606,0.0542,0.012,0.0422,0.0542,0.0422,0.012,0.0482,0.0181,0.0422,0.0542,0.0361,0.0542,0.0482,0.0181,0.012,0.0542,0.012,0.0542,0.0181,0.0301,0.0361,0.0181,0.0361,0.012,0.012,0.012]  Seed=50510
  read_ProcessTimer : ReadTimer  TimerTag=T_Process_17  StatAverageTimeElapsed=on
      settings: OutputPortMap=o3
  setRouting : SetAttribute  AttributeName=outputFlowNode  AttributeFrom=Signal port  EvaluatedAttributeValue={ []}
  start_ProcessTimer : StartTimer  TimerTag=T_Process_17  TimerStartedOption=Restart
  IN_Job : PMIOPort  Port=1  Side=Left
  OUT_Job : PMIOPort  Port=2  Side=Right
  wires:
  Routing/1 -> setRouting/1
  ProcessTime/1 -> ProcessServer/1
  connections:
  setRouting/LConn1 -- OUTQueue/RConn1
  IN_Job/RConn1 -- start_ProcessTimer/LConn1
  ProcessServer/RConn1 -- read_ProcessTimer/LConn1
  start_ProcessTimer/RConn1 -- ProcessQueue/LConn1
  ProcessQueue/RConn1 -- ProcessServer/LConn1
  read_ProcessTimer/RConn1 -- OUTQueue/LConn1
  OUT_Job/RConn1 -- setRouting/RConn1

== system ProcessNetworkSimulation/Process_18/Process ==
  OUTQueue : FIFOQueue  Capacity=inf
  ProcessQueue : FIFOQueue  Capacity=Inf  StatAverageWait=on  StatAverageQueueLength=on
      settings: OutputPortMap=o2,o3
  ProcessServer : NServer  NumberOfServers=11  ServiceTimeFrom=Signal port t  StatNumberDeparted=on  StatUtilization=on
      settings: OutputPortMap=o0,o5
  ProcessTime : EventBasedRandomNumber  meanExp=0.05  minUnif=1  meanNorm=2  stdNorm=0.2  Seed=53727
  Routing : EventBasedRandomNumber  Distribution=Arbitrary discrete  valueVecDisc=[0,1,2,3,4,5,6,7,8,9,10,11,12,13,14,15,16,17,18,19,20,21,22,23,24,25,26,27,28,29,30,31,32,33,34,35,36,37]  probVecDisc=[0,0.0055,0.0273,0.0548,0.0055,0.0164,0.0109,0.0492,0.0109,0.0109,0.0164,0.0273,0.0328,0.0383,0.0109,0.0273,0.0273,0.0546,0.0492,0.0273,0.0492,0.0109,0.0109,0.0437,0.0492,0.0328,0.0109,0.0273,0.0109,0.0109,0.0492,0.0492,0.0383,0.0273,0.0383,0.0273,0.0109,0]  Seed=56944
  read_ProcessTimer : ReadTimer  TimerTag=T_Process_18  StatAverageTimeElapsed=on
      settings: OutputPortMap=o3
  setRouting : SetAttribute  AttributeName=outputFlowNode  AttributeFrom=Signal port  EvaluatedAttributeValue={ []}
  start_ProcessTimer : StartTimer  TimerTag=T_Process_18  TimerStartedOption=Restart
  IN_Job : PMIOPort  Port=1  Side=Left
  OUT_Job : PMIOPort  Port=2  Side=Right
  wires:
  Routing/1 -> setRouting/1
  ProcessTime/1 -> ProcessServer/1
  connections:
  setRouting/LConn1 -- OUTQueue/RConn1
  IN_Job/RConn1 -- start_ProcessTimer/LConn1
  ProcessServer/RConn1 -- read_ProcessTimer/LConn1
  start_ProcessTimer/RConn1 -- ProcessQueue/LConn1
  ProcessQueue/RConn1 -- ProcessServer/LConn1
  read_ProcessTimer/RConn1 -- OUTQueue/LConn1
  OUT_Job/RConn1 -- setRouting/RConn1

== system ProcessNetworkSimulation/Process_19/Process ==
  OUTQueue : FIFOQueue  Capacity=inf
  ProcessQueue : FIFOQueue  Capacity=Inf  StatAverageWait=on  StatAverageQueueLength=on
      settings: OutputPortMap=o2,o3
  ProcessServer : NServer  NumberOfServers=12  ServiceTimeFrom=Signal port t  StatNumberDeparted=on  StatUtilization=on
      settings: OutputPortMap=o0,o5
  ProcessTime : EventBasedRandomNumber  meanExp=0.05  minUnif=1  meanNorm=2  stdNorm=0.2  Seed=60161
  Routing : EventBasedRandomNumber  Distribution=Arbitrary discrete  valueVecDisc=[0,1,2,3,4,5,6,7,8,9,10,11,12,13,14,15,16,17,18,19,20,21,22,23,24,25,26,27,28,29,30,31,32,33,34,35,36,37,38,39,40,41,42]  probVecDisc=[0,0.0367,0.0082,0.0367,0.0406,0.0367,0.0122,0.0286,0.0245,0.0082,0.0245,0.0408,0.0245,0.0082,0.0082,0.0286,0.0367,0.0286,0.0245,0.0245,0.0367,0.0245,0.0367,0.0245,0.0041,0.0286,0.0367,0.0082,0.0245,0.0082,0.0082,0.0286,0.0327,0.0367,0.0122,0.0367,0.0245,0.0286,0.0041,0.0082,0.0367,0.0286,0]  Seed=63378
  read_ProcessTimer : ReadTimer  TimerTag=T_Process_19  StatAverageTimeElapsed=on
      settings: OutputPortMap=o3
  setRouting : SetAttribute  AttributeName=outputFlowNode  AttributeFrom=Signal port  EvaluatedAttributeValue={ []}
  start_ProcessTimer : StartTimer  TimerTag=T_Process_19  TimerStartedOption=Restart
  IN_Job : PMIOPort  Port=1  Side=Left
  OUT_Job : PMIOPort  Port=2  Side=Right
  wires:
  Routing/1 -> setRouting/1
  ProcessTime/1 -> ProcessServer/1
  connections:
  setRouting/LConn1 -- OUTQueue/RConn1
  IN_Job/RConn1 -- start_ProcessTimer/LConn1
  ProcessServer/RConn1 -- read_ProcessTimer/LConn1
  start_ProcessTimer/RConn1 -- ProcessQueue/LConn1
  ProcessQueue/RConn1 -- ProcessServer/LConn1
  read_ProcessTimer/RConn1 -- OUTQueue/LConn1
  OUT_Job/RConn1 -- setRouting/RConn1

== system ProcessNetworkSimulation/Process_2/Process ==
  OUTQueue : FIFOQueue  Capacity=inf
  ProcessQueue : FIFOQueue  Capacity=Inf  StatAverageWait=on  StatAverageQueueLength=on
      settings: OutputPortMap=o2,o3
  ProcessServer : NServer  NumberOfServers=8  ServiceTimeFrom=Signal port t  StatNumberDeparted=on  StatUtilization=on
      settings: OutputPortMap=o0,o5
  ProcessTime : EventBasedRandomNumber  meanExp=0.05  minUnif=1  meanNorm=2  stdNorm=0.2  Seed=1059
  Routing : EventBasedRandomNumber  Distribution=Arbitrary discrete  valueVecDisc=[0,1,2,3,4,5,6,7,8,9,10,11,12,13,14,15,16,17,18,19,20,21,22,23,24,25,26,27,28,29,30,31,32]  probVecDisc=[0,0.0139,0.0417,0.0139,0.0626,0.0417,0.0486,0.0486,0.0139,0.0139,0.0486,0.0069,0.0208,0.0069,0.0139,0.0069,0.0486,0.0139,0.0625,0.0556,0.0347,0.0486,0.0208,0.0417,0.0347,0.0139,0.0486,0.0347,0.0625,0.0139,0.0486,0.0139,0]  Seed=7493
  read_ProcessTimer : ReadTimer  TimerTag=T_Process_2  StatAverageTimeElapsed=on
      settings: OutputPortMap=o3
  setRouting : SetAttribute  AttributeName=outputFlowNode  AttributeFrom=Signal port  EvaluatedAttributeValue={ []}
  start_ProcessTimer : StartTimer  TimerTag=T_Process_2  TimerStartedOption=Restart
  IN_Job : PMIOPort  Port=1  Side=Left
  OUT_Job : PMIOPort  Port=2  Side=Right
  wires:
  Routing/1 -> setRouting/1
  ProcessTime/1 -> ProcessServer/1
  connections:
  setRouting/LConn1 -- OUTQueue/RConn1
  IN_Job/RConn1 -- start_ProcessTimer/LConn1
  ProcessServer/RConn1 -- read_ProcessTimer/LConn1
  start_ProcessTimer/RConn1 -- ProcessQueue/LConn1
  ProcessQueue/RConn1 -- ProcessServer/LConn1
  read_ProcessTimer/RConn1 -- OUTQueue/LConn1
  OUT_Job/RConn1 -- setRouting/RConn1

== system ProcessNetworkSimulation/Process_20/Process ==
  OUTQueue : FIFOQueue  Capacity=inf
  ProcessQueue : FIFOQueue  Capacity=Inf  StatAverageWait=on  StatAverageQueueLength=on
      settings: OutputPortMap=o2,o3
  ProcessServer : NServer  NumberOfServers=12  ServiceTimeFrom=Signal port t  StatNumberDeparted=on  StatUtilization=on
      settings: OutputPortMap=o0,o5
  ProcessTime : EventBasedRandomNumber  meanExp=0.05  minUnif=1  meanNorm=2  stdNorm=0.2  Seed=10710
  Routing : EventBasedRandomNumber  Distribution=Arbitrary discrete  valueVecDisc=[0,1,2,3,4,5,6,7,8,9,10,11,12,13,14,15,16,17,18,19,20,21,22,23,24,25,26,27,28,29,30,31,32,33,34,35,36,37,38,39,40,41,42]  probVecDisc=[0,0.0078,0.0078,0.0271,0.0271,0.0233,0.0078,0.0233,0.0349,0.0271,0.0349,0.0078,0.0349,0.0271,0.0349,0.0349,0.0381,0.0271,0.0078,0.0078,0.0233,0.0271,0.0271,0.0271,0.0233,0.0349,0.0194,0.0078,0.0349,0.031,0.0233,0.0078,0.0388,0.0233,0.0233,0.0078,0.0349,0.0271,0.0349,0.0349,0.0349,0.0116,0]  Seed=13927
  read_ProcessTimer : ReadTimer  TimerTag=T_Process_20  StatAverageTimeElapsed=on
      settings: OutputPortMap=o3
  setRouting : SetAttribute  AttributeName=outputFlowNode  AttributeFrom=Signal port  EvaluatedAttributeValue={ []}
  start_ProcessTimer : StartTimer  TimerTag=T_Process_20  TimerStartedOption=Restart
  IN_Job : PMIOPort  Port=1  Side=Left
  OUT_Job : PMIOPort  Port=2  Side=Right
  wires:
  Routing/1 -> setRouting/1
  ProcessTime/1 -> ProcessServer/1
  connections:
  setRouting/LConn1 -- OUTQueue/RConn1
  IN_Job/RConn1 -- start_ProcessTimer/LConn1
  ProcessServer/RConn1 -- read_ProcessTimer/LConn1
  start_ProcessTimer/RConn1 -- ProcessQueue/LConn1
  ProcessQueue/RConn1 -- ProcessServer/LConn1
  read_ProcessTimer/RConn1 -- OUTQueue/LConn1
  OUT_Job/RConn1 -- setRouting/RConn1

== system ProcessNetworkSimulation/Process_21/Process ==
  OUTQueue : FIFOQueue  Capacity=inf
  ProcessQueue : FIFOQueue  Capacity=Inf  StatAverageWait=on  StatAverageQueueLength=on
      settings: OutputPortMap=o2,o3
  ProcessServer : NServer  NumberOfServers=10  ServiceTimeFrom=Signal port t  StatNumberDeparted=on  StatUtilization=on
      settings: OutputPortMap=o0,o5
  ProcessTime : EventBasedRandomNumber  meanExp=0.05  minUnif=1  meanNorm=2  stdNorm=0.2  Seed=17144
  Routing : EventBasedRandomNumber  Distribution=Arbitrary discrete  valueVecDisc=[0,1,2,3,4,5,6,7,8,9,10,11,12,13,14,15,16,17,18,19,20,21,22,23,24,25,26,27,28,29,30,31,32,33,34]  probVecDisc=[0,0.0376,0.0269,0.0161,0.0376,0.0376,0.0161,0.043,0.0323,0.0269,0.0376,0.0108,0.0108,0.0537,0.0269,0.0323,0.0108,0.0269,0.0484,0.0376,0.0376,0.0108,0.0108,0.0376,0.0269,0.0484,0.0376,0.0538,0.0161,0.0376,0.0484,0.0161,0.0108,0.0376,0]  Seed=20361
  read_ProcessTimer : ReadTimer  TimerTag=T_Process_21  StatAverageTimeElapsed=on
      settings: OutputPortMap=o3
  setRouting : SetAttribute  AttributeName=outputFlowNode  AttributeFrom=Signal port  EvaluatedAttributeValue={ []}
  start_ProcessTimer : StartTimer  TimerTag=T_Process_21  TimerStartedOption=Restart
  IN_Job : PMIOPort  Port=1  Side=Left
  OUT_Job : PMIOPort  Port=2  Side=Right
  wires:
  Routing/1 -> setRouting/1
  ProcessTime/1 -> ProcessServer/1
  connections:
  setRouting/LConn1 -- OUTQueue/RConn1
  IN_Job/RConn1 -- start_ProcessTimer/LConn1
  ProcessServer/RConn1 -- read_ProcessTimer/LConn1
  start_ProcessTimer/RConn1 -- ProcessQueue/LConn1
  ProcessQueue/RConn1 -- ProcessServer/LConn1
  read_ProcessTimer/RConn1 -- OUTQueue/LConn1
  OUT_Job/RConn1 -- setRouting/RConn1
